simulink model "DieukhienVOC_PWM"  (R2020b)
settings: Solver=FixedStepAuto  StartTime=0.0  StopTime=8  FixedStep=2e-6  RelTol=1e-3
values from neighbouring files (symbols this model uses):
  C = 10000e-6    (= 0.01)    [thongso.m]
  L = 2e-3    (= 0.002)    [thongso.m]
  R = 0.1    [thongso.m]
  Rload = 20    [thongso.m]
libraries: powerlib x11, pid_lib x3
settings Model: Creator=chemi  LastModifiedBy=chemi

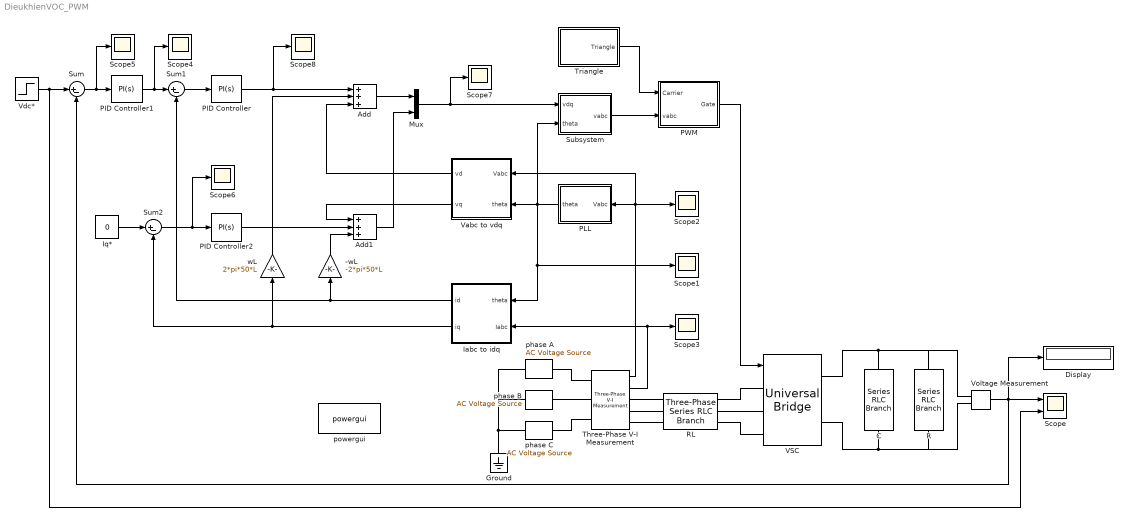
== system DieukhienVOC_PWM ==
  -wL : Gain  Gain=-2*pi*50*L
  Add : Sum  Inputs=+++
  Add1 : Sum  Inputs=+++
  C : powerlib/Elements/Series RLC Branch  LConnTagsString=__new0  RConnTagsString=__new0  BranchType=C  Resistance=1  Inductance=1e-3  SetiL0=off  InitialCurrent=0  Capacitance=C  Setx0=off  InitialVoltage=0  Measurements=None
  Display : Display
  Ground : powerlib/Elements/Ground  LConnTagsString=a
  Iabc to idq : Subsystem
  Iq* : Constant  Value=0
  Mux : Mux  Inputs=2
  PID Controller : pid_lib/PID Controller  Controller=PI  Form=Parallel  TimeDomain=Continuous-time  UseExternalTs=off  SampleTime=-1  IntegratorMethod=Forward Euler  FilterMethod=Forward Euler  ControllerParametersSource=internal  P=2000  I=100  D=0  UseFilter=on  N=100  TunerSelectOption=Transfer Function Based (PID Tuner App)  InitialConditionSource=internal  InitialConditionForIntegrator=0  InitialConditionForFilter=0  DifferentiatorICPrevScaledInput=0  ExternalReset=none  TrackingMode=off  Kt=1  LimitOutput=off  SatLimitsSource=internal  UpperSaturationLimit=inf  LowerSaturationLimit=-inf  LinearizeAsGain=on  AntiWindupMode=none  Kb=1  POutMin=[]  POutMax=[]  IOutMin=[]  IOutMax=[]  DOutMin=[]  DOutMax=[]  NOutMin=[]  NOutMax=[]  SumOutMin=[]  SumOutMax=[]  SaturationOutMin=[]  SaturationOutMax=[]  PParamMin=[]  PParamMax=[]  IParamMin=[]  IParamMax=[]  DParamMin=[]  DParamMax=[]  NParamMin=[]  NParamMax=[]  KbParamMin=[]  KbParamMax=[]  KtParamMin=[]  KtParamMax=[]  KbOutMin=[]  KbOutMax=[]  KtOutMin=[]  KtOutMax=[]  IntegratorOutMin=[]  IntegratorOutMax=[]  FilterOutMin=[]  FilterOutMax=[]  SumI1OutMin=[]  SumI1OutMax=[]  SumI2OutMin=[]  SumI2OutMax=[]  SumI3OutMin=[]  SumI3OutMax=[]  SumI4OutMin=[]  SumI4OutMax=[]  SumDOutMin=[]  SumDOutMax=[]  DifferentiatorOutMin=[]  DifferentiatorOutMax=[]  FilterDiffOutCoefMin=[]  FilterDiffOutCoefMax=[]  ReciprocalOutMin=[]  ReciprocalOutMax=[]  SumDenOutMin=[]  SumDenOutMax=[]  SumNumOutMin=[]  SumNumOutMax=[]  DivideOutMin=[]  DivideOutMax=[]  UdiffTsProdOutMin=[]  UdiffTsProdOutMax=[]  NTsProdOutMin=[]  NTsProdOutMax=[]  UintegralTsProdOutMin=[]  UintegralTsProdOutMax=[]  UngainTsProdOutMin=[]  UngainTsProdOutMax=[]  IntegratorContinuousStateAttributes=''  IntegratorStateMustResolveToSignalObject=off  IntegratorRTWStateStorageClass=Auto  FilterContinuousStateAttributes=''  FilterStateMustResolveToSignalObject=off  FilterRTWStateStorageClass=Auto  ParallelPVariant=InternalParameters  IdealPVariant=Disabled  IVariant=InternalParameters  DVariant=Disabled  IntegratorVariant=Continuous  SatVariant=Disabled  AWVariant=Passthrough  PCopyVariant=Disabled  TRVariant=Disabled  FdbkBlocksVariant=Forward  IdealPFdbkVariant=Disabled  SatFdbkVariant=Disabled  DerivativeFilterVariant=Disabled  NVariant=Disabled  NCopyVariant=Disabled_SignalSpec  FilterICVariant=Disabled  IntegratorICVariant=InternalICs  ExternalResetVariant=Disabled  TRSumVariant=Passthrough  SumFdbkVariant=Disabled  SumVariant=Sum_PI  TsampFilterVariant=InternalTs  TsampNgainVariant=Passthrough  TsampIntegralVariant=Passthrough  ExternalSaturationOutDataTypeStr=Inherit: Same as second input
  PID Controller1 : pid_lib/PID Controller  Controller=PI  Form=Parallel  TimeDomain=Continuous-time  UseExternalTs=off  SampleTime=-1  IntegratorMethod=Forward Euler  FilterMethod=Forward Euler  ControllerParametersSource=internal  P=5  I=50  D=0  UseFilter=on  N=100  TunerSelectOption=Transfer Function Based (PID Tuner App)  InitialConditionSource=internal  InitialConditionForIntegrator=0  InitialConditionForFilter=0  DifferentiatorICPrevScaledInput=0  ExternalReset=none  TrackingMode=off  Kt=1  LimitOutput=off  SatLimitsSource=internal  UpperSaturationLimit=inf  LowerSaturationLimit=-inf  LinearizeAsGain=on  AntiWindupMode=none  Kb=1  POutMin=[]  POutMax=[]  IOutMin=[]  IOutMax=[]  DOutMin=[]  DOutMax=[]  NOutMin=[]  NOutMax=[]  SumOutMin=[]  SumOutMax=[]  SaturationOutMin=[]  SaturationOutMax=[]  PParamMin=[]  PParamMax=[]  IParamMin=[]  IParamMax=[]  DParamMin=[]  DParamMax=[]  NParamMin=[]  NParamMax=[]  KbParamMin=[]  KbParamMax=[]  KtParamMin=[]  KtParamMax=[]  KbOutMin=[]  KbOutMax=[]  KtOutMin=[]  KtOutMax=[]  IntegratorOutMin=[]  IntegratorOutMax=[]  FilterOutMin=[]  FilterOutMax=[]  SumI1OutMin=[]  SumI1OutMax=[]  SumI2OutMin=[]  SumI2OutMax=[]  SumI3OutMin=[]  SumI3OutMax=[]  SumI4OutMin=[]  SumI4OutMax=[]  SumDOutMin=[]  SumDOutMax=[]  DifferentiatorOutMin=[]  DifferentiatorOutMax=[]  FilterDiffOutCoefMin=[]  FilterDiffOutCoefMax=[]  ReciprocalOutMin=[]  ReciprocalOutMax=[]  SumDenOutMin=[]  SumDenOutMax=[]  SumNumOutMin=[]  SumNumOutMax=[]  DivideOutMin=[]  DivideOutMax=[]  UdiffTsProdOutMin=[]  UdiffTsProdOutMax=[]  NTsProdOutMin=[]  NTsProdOutMax=[]  UintegralTsProdOutMin=[]  UintegralTsProdOutMax=[]  UngainTsProdOutMin=[]  UngainTsProdOutMax=[]  IntegratorContinuousStateAttributes=''  IntegratorStateMustResolveToSignalObject=off  IntegratorRTWStateStorageClass=Auto  FilterContinuousStateAttributes=''  FilterStateMustResolveToSignalObject=off  FilterRTWStateStorageClass=Auto  ParallelPVariant=InternalParameters  IdealPVariant=Disabled  IVariant=InternalParameters  DVariant=Disabled  IntegratorVariant=Continuous  SatVariant=Disabled  AWVariant=Passthrough  PCopyVariant=Disabled  TRVariant=Disabled  FdbkBlocksVariant=Forward  IdealPFdbkVariant=Disabled  SatFdbkVariant=Disabled  DerivativeFilterVariant=Disabled  NVariant=Disabled  NCopyVariant=Disabled_SignalSpec  FilterICVariant=Disabled  IntegratorICVariant=InternalICs  ExternalResetVariant=Disabled  TRSumVariant=Passthrough  SumFdbkVariant=Disabled  SumVariant=Sum_PI  TsampFilterVariant=InternalTs  TsampNgainVariant=Passthrough  TsampIntegralVariant=Passthrough  ExternalSaturationOutDataTypeStr=Inherit: Same as second input
  PID Controller2 : pid_lib/PID Controller  Controller=PI  Form=Parallel  TimeDomain=Continuous-time  UseExternalTs=off  SampleTime=-1  IntegratorMethod=Forward Euler  FilterMethod=Forward Euler  ControllerParametersSource=internal  P=2000  I=100  D=0  UseFilter=on  N=100  TunerSelectOption=Transfer Function Based (PID Tuner App)  InitialConditionSource=internal  InitialConditionForIntegrator=0  InitialConditionForFilter=0  DifferentiatorICPrevScaledInput=0  ExternalReset=none  TrackingMode=off  Kt=1  LimitOutput=off  SatLimitsSource=internal  UpperSaturationLimit=inf  LowerSaturationLimit=-inf  LinearizeAsGain=on  AntiWindupMode=none  Kb=1  POutMin=[]  POutMax=[]  IOutMin=[]  IOutMax=[]  DOutMin=[]  DOutMax=[]  NOutMin=[]  NOutMax=[]  SumOutMin=[]  SumOutMax=[]  SaturationOutMin=[]  SaturationOutMax=[]  PParamMin=[]  PParamMax=[]  IParamMin=[]  IParamMax=[]  DParamMin=[]  DParamMax=[]  NParamMin=[]  NParamMax=[]  KbParamMin=[]  KbParamMax=[]  KtParamMin=[]  KtParamMax=[]  KbOutMin=[]  KbOutMax=[]  KtOutMin=[]  KtOutMax=[]  IntegratorOutMin=[]  IntegratorOutMax=[]  FilterOutMin=[]  FilterOutMax=[]  SumI1OutMin=[]  SumI1OutMax=[]  SumI2OutMin=[]  SumI2OutMax=[]  SumI3OutMin=[]  SumI3OutMax=[]  SumI4OutMin=[]  SumI4OutMax=[]  SumDOutMin=[]  SumDOutMax=[]  DifferentiatorOutMin=[]  DifferentiatorOutMax=[]  FilterDiffOutCoefMin=[]  FilterDiffOutCoefMax=[]  ReciprocalOutMin=[]  ReciprocalOutMax=[]  SumDenOutMin=[]  SumDenOutMax=[]  SumNumOutMin=[]  SumNumOutMax=[]  DivideOutMin=[]  DivideOutMax=[]  UdiffTsProdOutMin=[]  UdiffTsProdOutMax=[]  NTsProdOutMin=[]  NTsProdOutMax=[]  UintegralTsProdOutMin=[]  UintegralTsProdOutMax=[]  UngainTsProdOutMin=[]  UngainTsProdOutMax=[]  IntegratorContinuousStateAttributes=''  IntegratorStateMustResolveToSignalObject=off  IntegratorRTWStateStorageClass=Auto  FilterContinuousStateAttributes=''  FilterStateMustResolveToSignalObject=off  FilterRTWStateStorageClass=Auto  ParallelPVariant=InternalParameters  IdealPVariant=Disabled  IVariant=InternalParameters  DVariant=Disabled  IntegratorVariant=Continuous  SatVariant=Disabled  AWVariant=Passthrough  PCopyVariant=Disabled  TRVariant=Disabled  FdbkBlocksVariant=Forward  IdealPFdbkVariant=Disabled  SatFdbkVariant=Disabled  DerivativeFilterVariant=Disabled  NVariant=Disabled  NCopyVariant=Disabled_SignalSpec  FilterICVariant=Disabled  IntegratorICVariant=InternalICs  ExternalResetVariant=Disabled  TRSumVariant=Passthrough  SumFdbkVariant=Disabled  SumVariant=Sum_PI  TsampFilterVariant=InternalTs  TsampNgainVariant=Passthrough  TsampIntegralVariant=Passthrough  ExternalSaturationOutDataTypeStr=Inherit: Same as second input
  PLL : Subsystem
  PWM : Subsystem
  R : powerlib/Elements/Series RLC Branch  LConnTagsString=__new0  RConnTagsString=__new0  BranchType=R  Resistance=Rload  Inductance=1e-3  SetiL0=off  InitialCurrent=0  Capacitance=1e-6  Setx0=off  InitialVoltage=0  Measurements=None
  RL : powerlib/Elements/Three-Phase Series RLC Branch  LConnTagsString=A|B|C  RConnTagsString=A|B|C  BranchType=RL  Resistance=R  Inductance=L  Capacitance=1e-6  Measurements=None
  Scope : Scope  NumInputPorts=2
  Scope{1..8} (8 alike) : Scope
  Subsystem : Subsystem
  Sum : Sum  Inputs=|+-
  Sum1 : Sum  Inputs=|+-
  Sum2 : Sum  Inputs=|+-
  Three-Phase V-I Measurement : powerlib/Measurements/Three-Phase V-I Measurement  VoltageMeasurement=phase-to-ground  SetLabelV=off  LabelV=Vabc  Vpu=off  VpuLL=off  CurrentMeasurement=yes  SetLabelI=off  LabelI=Iabc  Ipu=off  Pbase=100e6  Vbase=500e3  OutputType=Complex  PhasorSimulation=off  PSBequivalent=0
  Triangle : Subsystem
  VSC : powerlib/Power Electronics/Universal Bridge  Arms=3  SnubberResistance=1e5  SnubberCapacitance=inf  Device=IGBT / Diodes  Ron=1e-3  Lon=0  ForwardVoltages="[  0  0  ]"  ForwardVoltage=0  GTOparameters=[ 10e-6 , 20e-6 ]  IGBTparameters=[ 1e-6 , 2e-6 ]  Measurements=None  Measurements_2=None  converterType=Rectifier
  Vabc to vdq : Subsystem
  Vdc* : Step  Time=0.5  After=200  SampleTime=0
  Voltage Measurement : powerlib/Measurements/Voltage Measurement  PhasorSimulation=off  OutputType=Complex  PSBequivalent=0
  phase A : powerlib/Electrical Sources/AC Voltage Source  Amplitude=220*sqrt(2)  Phase=0  Frequency=50  SampleTime=0  Measurements=None  BusType=swing  Pref=10e3  Qref=0  Qmin=-inf  Qmax=+inf
  phase B : powerlib/Electrical Sources/AC Voltage Source  Amplitude=220*sqrt(2)  Phase=120  Frequency=50  SampleTime=0  Measurements=None  BusType=swing  Pref=10e3  Qref=0  Qmin=-inf  Qmax=+inf
  phase C : powerlib/Electrical Sources/AC Voltage Source  Amplitude=220*sqrt(2)  Phase=240  Frequency=50  SampleTime=0  Measurements=None  BusType=swing  Pref=10e3  Qref=0  Qmin=-inf  Qmax=+inf
  powergui : powerlib/powergui  Priority=1  SimulationMode=Discrete  SampleTime=2e-6  frequency=60  Iterations=50  frequencyindice=50  Pbase=100e6  ErrMax=1e-4  UnitsV=kV  UnitsW=MW  buscounter=0  FunctionMessages=off  echomessages=off  EnableUseOfTLC=off  CurrentSourceSwitches=off  DisableSnubberDevices=off  DisableRonSwitches=off  DisableVfSwitches=off  DisplayEquations=off  AutomaticDiscreteSolvers=off  SolverType=Tustin/Backward Euler (TBE)  Interpol=off  ExternalGateDelay=off  methode=off  Ts=100  x0status=blocks  SPID=on  SwTol=0  HookPort=off  NonlinearTolerance=1e-4  nMaxIteration=100  ContinueOnMaxIteration=off  RestoreLinks=warning  ResistiveCurrentMeasurement=off  Frange=[0:2:500]  Ylog=off  Xlog=on  ShowGrid=off  save=off  variable=ZData  structure=0  ZoomFFT=off  StartTime=0.0  cycles=1  DisplayStyle=1  fundamental=60  FreqAxis=off  MaxFrequency=1000  frequencyindicesteady=1  RmsSteady=1  display=off
  wL : Gain  Gain=2*pi*50*L
  wires:
  Three-Phase V-I Measurement/1 -> Scope2/1, Vabc to vdq/1(Vabc), PLL/1(Vabc)
  PLL/1(theta) -> Scope1/1, Iabc to idq/1(theta), Subsystem/2(theta), Vabc to vdq/2(theta)
  Three-Phase V-I Measurement/2 -> Iabc to idq/2(Iabc), Scope3/1
  Vdc*/1 -> Scope/2, Sum/1
  Sum/1 -> Scope5/1, PID Controller1/1
  PID Controller1/1 -> Scope4/1, Sum1/1
  Iabc to idq/1(id) -> -wL/1, Sum1/2
  Iabc to idq/2(iq) -> Sum2/2, wL/1
  Iq*/1 -> Sum2/1
  Sum1/1 -> PID Controller/1
  Sum2/1 -> Scope6/1, PID Controller2/1
  PID Controller/1 -> Scope8/1, Add/1
  wL/1 -> Add/2
  PID Controller2/1 -> Add1/2
  -wL/1 -> Add1/3
  Add/1 -> Mux/1
  Add1/1 -> Mux/2
  Voltage Measurement/1 -> Display/1, Scope/1, Sum/2
  PWM/1(Gate) -> VSC/1
  Triangle/1(Triangle) -> PWM/1(Carrier)
  Vabc to vdq/1(vd) -> Add/3
  Vabc to vdq/2(vq) -> Add1/1
  Mux/1 -> Scope7/1, Subsystem/1(vdq)
  Subsystem/1(vabc) -> PWM/2(vabc)
  connections:
  Ground/LConn1 -- phase A/LConn1 -- phase B/LConn1 -- phase C/LConn1
  phase A/RConn1 -- Three-Phase V-I Measurement/LConn1
  phase B/RConn1 -- Three-Phase V-I Measurement/LConn2
  phase C/RConn1 -- Three-Phase V-I Measurement/LConn3
  RL/LConn1 -- Three-Phase V-I Measurement/RConn1
  RL/LConn2 -- Three-Phase V-I Measurement/RConn2
  RL/LConn3 -- Three-Phase V-I Measurement/RConn3
  VSC/LConn2 -- RL/RConn2
  RL/RConn1 -- VSC/LConn1
  RL/RConn3 -- VSC/LConn3
  VSC/RConn1 -- C/LConn1 -- Voltage Measurement/LConn1 -- R/LConn1
  VSC/RConn2 -- Voltage Measurement/LConn2 -- R/RConn1 -- C/RConn1

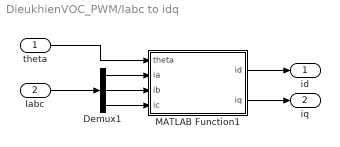
== system DieukhienVOC_PWM/Iabc to idq ==
  theta : Inport
  Iabc : Inport  Port=2
  Demux1 : Demux  Outputs=3
  MATLAB Function1 : MATLAB Function  TreatAsAtomicUnit=on
  id : Outport  VectorParamsAs1DForOutWhenUnconnected=off
  iq : Outport  Port=2  VectorParamsAs1DForOutWhenUnconnected=off
  wires:
  Iabc/1 -> Demux1/1
  Demux1/1 -> MATLAB Function1/2(ia)
  Demux1/2 -> MATLAB Function1/3(ib)
  Demux1/3 -> MATLAB Function1/4(ic)
  theta/1 -> MATLAB Function1/1(theta)
  MATLAB Function1/2(iq) -> iq/1
  MATLAB Function1/1(id) -> id/1

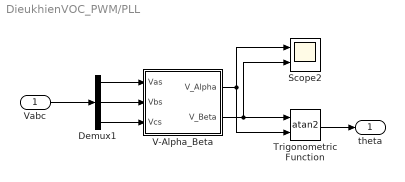
== system DieukhienVOC_PWM/PLL ==
  Vabc : Inport
  Demux1 : Demux  Outputs=3
  Scope2 : Scope  NumInputPorts=2
  Trigonometric Function : Trigonometry  Operator=atan2
  V-Alpha_Beta : Subsystem
  theta : Outport
  wires:
  Vabc/1 -> Demux1/1
  Demux1/2 -> V-Alpha_Beta/2(Vbs)
  Demux1/1 -> V-Alpha_Beta/1(Vas)
  Demux1/3 -> V-Alpha_Beta/3(Vcs)
  V-Alpha_Beta/1(V_Alpha) -> Trigonometric Function/2, Scope2/1
  V-Alpha_Beta/2(V_Beta) -> Scope2/2, Trigonometric Function/1
  Trigonometric Function/1 -> theta/1

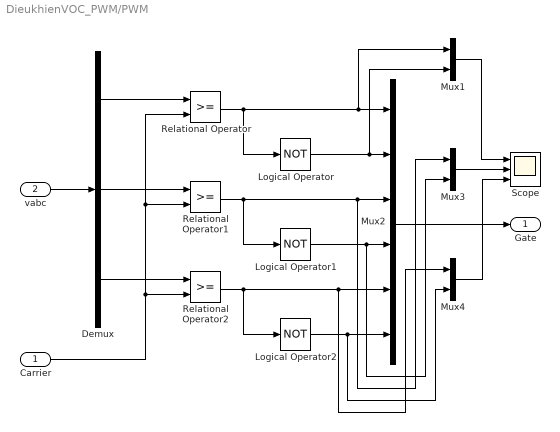
== system DieukhienVOC_PWM/PWM ==
  Carrier : Inport
  vabc : Inport  Port=2
  Demux : Demux  Outputs=3
  Logical Operator : Logic  Operator=NOT  AllPortsSameDT=off  OutDataTypeStr=boolean
  Logical Operator1 : Logic  Operator=NOT  AllPortsSameDT=off  OutDataTypeStr=boolean
  Logical Operator2 : Logic  Operator=NOT  AllPortsSameDT=off  OutDataTypeStr=boolean
  Mux1 : Mux  Inputs=2
  Mux2 : Mux  Inputs=6
  Mux3 : Mux  Inputs=2
  Mux4 : Mux  Inputs=2
  Relational Operator : RelationalOperator  OutDataTypeStr=boolean  RndMeth=Simplest
  Relational Operator1 : RelationalOperator  OutDataTypeStr=boolean  RndMeth=Simplest
  Relational Operator2 : RelationalOperator  OutDataTypeStr=boolean  RndMeth=Simplest
  Scope : Scope  NumInputPorts=3
  Gate : Outport
  wires:
  vabc/1 -> Demux/1
  Demux/1 -> Relational Operator/1
  Mux2/1 -> Gate/1
  Relational Operator/1 -> Logical Operator/1, Mux1/1, Mux2/1
  Logical Operator/1 -> Mux1/2, Mux2/2
  Carrier/1 -> Relational Operator2/2, Relational Operator1/2, Relational Operator/2
  Relational Operator1/1 -> Logical Operator1/1, Mux3/1, Mux2/3
  Logical Operator1/1 -> Mux3/2, Mux2/4
  Demux/2 -> Relational Operator1/1
  Logical Operator2/1 -> Mux4/2, Mux2/6
  Relational Operator2/1 -> Mux4/1, Mux2/5, Logical Operator2/1
  Demux/3 -> Relational Operator2/1
  Mux1/1 -> Scope/1
  Mux3/1 -> Scope/2
  Mux4/1 -> Scope/3

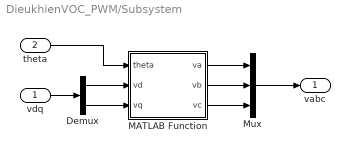
== system DieukhienVOC_PWM/Subsystem ==
  vdq : Inport
  theta : Inport  Port=2
  Demux : Demux  Outputs=2
  MATLAB Function : MATLAB Function  TreatAsAtomicUnit=on
  Mux : Mux  Inputs=3
  vabc : Outport
  wires:
  Demux/1 -> MATLAB Function/2(vd)
  Demux/2 -> MATLAB Function/3(vq)
  theta/1 -> MATLAB Function/1(theta)
  vdq/1 -> Demux/1
  MATLAB Function/1(va) -> Mux/1
  MATLAB Function/2(vb) -> Mux/2
  MATLAB Function/3(vc) -> Mux/3
  Mux/1 -> vabc/1

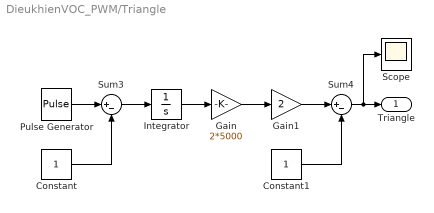
== system DieukhienVOC_PWM/Triangle ==
  Constant : Constant
  Constant1 : Constant
  Gain : Gain  Gain=2*5000
  Gain1 : Gain  Gain=2
  Integrator : Integrator
  Pulse Generator : DiscretePulseGenerator  PulseType=Time based  Amplitude=2  Period=1/5000  PulseWidth=50  PhaseDelay=2e-6
  Scope : Scope
  Sum3 : Sum  Inputs=|+-
  Sum4 : Sum  Inputs=|+-
  Triangle : Outport
  wires:
  Integrator/1 -> Gain/1
  Constant1/1 -> Sum4/2
  Constant/1 -> Sum3/2
  Sum3/1 -> Integrator/1
  Gain1/1 -> Sum4/1
  Pulse Generator/1 -> Sum3/1
  Sum4/1 -> Scope/1, Triangle/1
  Gain/1 -> Gain1/1

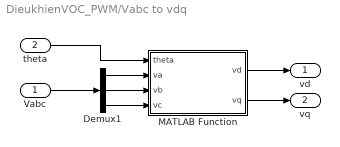
== system DieukhienVOC_PWM/Vabc to vdq ==
  Vabc : Inport
  theta : Inport  Port=2
  Demux1 : Demux  Outputs=3
  MATLAB Function : MATLAB Function  TreatAsAtomicUnit=on
  vd : Outport  VectorParamsAs1DForOutWhenUnconnected=off
  vq : Outport  Port=2  VectorParamsAs1DForOutWhenUnconnected=off
  wires:
  theta/1 -> MATLAB Function/1(theta)
  Demux1/3 -> MATLAB Function/4(vc)
  Demux1/2 -> MATLAB Function/3(vb)
  Demux1/1 -> MATLAB Function/2(va)
  Vabc/1 -> Demux1/1
  MATLAB Function/1(vd) -> vd/1
  MATLAB Function/2(vq) -> vq/1

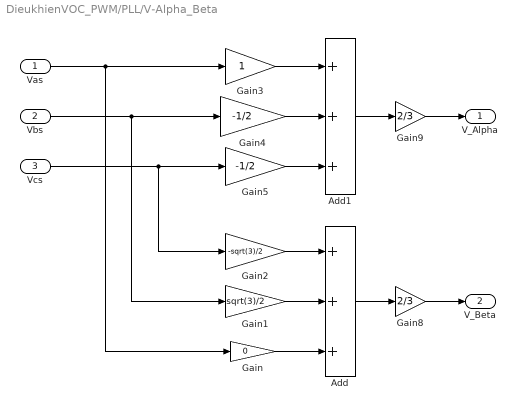
== system DieukhienVOC_PWM/PLL/V-Alpha_Beta ==
  Vas : Inport
  Vbs : Inport  Port=2
  Vcs : Inport  Port=3
  Add : Sum  Inputs=+++
  Add1 : Sum  Inputs=+++
  Gain : Gain  Gain=0
  Gain1 : Gain  Gain=sqrt(3)/2
  Gain2 : Gain  Gain=-sqrt(3)/2
  Gain3 : Gain
  Gain4 : Gain  Gain=-1/2
  Gain5 : Gain  Gain=-1/2
  Gain8 : Gain  Gain=2/3
  Gain9 : Gain  Gain=2/3
  V_Alpha : Outport  VectorParamsAs1DForOutWhenUnconnected=off
  V_Beta : Outport  Port=2  VectorParamsAs1DForOutWhenUnconnected=off
  wires:
  Vbs/1 -> Gain1/1, Gain4/1
  Vas/1 -> Gain/1, Gain3/1
  Gain5/1 -> Add1/3
  Vcs/1 -> Gain2/1, Gain5/1
  Gain4/1 -> Add1/2
  Gain3/1 -> Add1/1
  Add/1 -> Gain8/1
  Add1/1 -> Gain9/1
  Gain8/1 -> V_Beta/1
  Gain9/1 -> V_Alpha/1
  Gain2/1 -> Add/1
  Gain1/1 -> Add/2
  Gain/1 -> Add/3

== matlab function DieukhienVOC_PWM/Subsystem/MATLAB Function ==
  data: theta input; vd input; vq input; va output; vb output; vc output
function [va,vb,vc] = fcn(theta,vd,vq)
va = vd*cos(theta)-vq*sin(theta);
vb = vd*cos(theta-2*pi/3)-vq*sin(theta-2*pi/3);
vc = vd*cos(theta+2*pi/3)-vq*sin(theta+2*pi/3);

== matlab function DieukhienVOC_PWM/Vabc to vdq/MATLAB Function ==
  data: theta input; va input; vb input; vd output; vc input; vq output
function [vd,vq] =   fcn(theta,va,vb,vc)
vd = (va*cos(theta)+vb*cos(theta-2*pi/3)+vc*cos(theta+2*pi/3))*2/3;
vq = (-va*sin(theta)-vb*sin(theta-2*pi/3)-vc*sin(theta+2*pi/3))*2/3;

== matlab function DieukhienVOC_PWM/Iabc to idq/MATLAB Function1 ==
  data: theta input; ia input; ib input; id output; ic input; iq output
function [id,iq] =   fcn(theta,ia,ib,ic)
id = (ia*cos(theta)+ib*cos(theta-2*pi/3)+ic*cos(theta+2*pi/3))*2/3;
iq = (-ia*sin(theta)-ib*sin(theta-2*pi/3)-ic*sin(theta+2*pi/3))*2/3;
